simulink model "building_PHPP_v2"  (R2023b)
settings: Solver=ode23s  StartTime=-building.preruntime+8760*3600  StopTime=building.runtime+8760*3600  EnableMultiTasking=on
PreLoadFcn:
  | tic
StartFcn:
  | pre_time = toc
  | assignin('base','pre_time',pre_time)
  | tic
StopFcn:
  | time = toc
  | assignin('base','time',time)
values from neighbouring files (symbols this model uses):
  building = obj    [BUILDING.m]    (also in create_building_automatic.m = building.save(); ini_building_automatic.m = building.add_variant_hvac(building.variant_hvac, hvac); load_building_automatic.m = building.save())
  cp = str2num(value)    [CONSTRUCTION.m]
  p = [timevec_weather weather(:,12)]    [BOUNDARY.m]    (also in WEATHER.m = 0; init_carnotUIBK.m = cell2mat(carnotUIBKpaths(i,2)))
  rho = str2num(value)    [CONSTRUCTION.m]    (also in theta_ground_v1.m = 2000)
undefined symbols (not defined in the file or in its folder): Dreifach, get_building, Qdot_C, Qdot_C_energy, Qdot_H, Qdot_H_energy, Qdot_I_electricity, Qdot_I_electricity_energy, Qdot_I_light, Qdot_I_light_energy, Qdot_I_person, Qdot_I_person_energy, Qdot_S, Qdot_S_energy, Qdot_T_ground, Qdot_T_ground_energy, Qdot_T_neighbour, Qdot_T_neighbour_energy, Qdot_T_opaque, Qdot_T_opaque_energy, Qdot_T_window, Qdot_T_window_energy, Qdot_V_infiltration, Qdot_V_infiltration_energy, Qdot_V_mech, Qdot_V_mech_energy, Qdot_V_window, Qdot_V_window_energy, Tc, Tr, Ts, Wärmeschutzglas, x_CO2, x_H2O, x_VOC
libraries: carnotUIBK x2418, carnot x1
(part 32 of 32)

== system building_PHPP_v2/DATALOGGER/logger_BDB/z4/Subsystem11 ==
  In1 : Inport
  Integrator1 : Integrator
  Ws->kWh : Gain  Gain=1/3600/1000
  Out1 : Outport  VectorParamsAs1DForOutWhenUnconnected=off
  wires:
  Ws->kWh/1 -> Out1/1
  Integrator1/1 -> Ws->kWh/1
  In1/1 -> Integrator1/1

== system building_PHPP_v2/DATALOGGER/logger_BDB/z4/Subsystem12 ==
  In1 : Inport
  Integrator1 : Integrator
  Ws->kWh : Gain  Gain=1/3600/1000
  Out1 : Outport  VectorParamsAs1DForOutWhenUnconnected=off
  wires:
  In1/1 -> Integrator1/1
  Integrator1/1 -> Ws->kWh/1
  Ws->kWh/1 -> Out1/1

== system building_PHPP_v2/DATALOGGER/logger_BDB/z4/Subsystem2 ==
  In1 : Inport
  Integrator1 : Integrator
  Ws->kWh : Gain  Gain=1/3600/1000
  Out1 : Outport  VectorParamsAs1DForOutWhenUnconnected=off
  wires:
  In1/1 -> Integrator1/1
  Integrator1/1 -> Ws->kWh/1
  Ws->kWh/1 -> Out1/1

== system building_PHPP_v2/DATALOGGER/logger_BDB/z4/Subsystem3 ==
  In1 : Inport
  Integrator1 : Integrator
  Ws->kWh : Gain  Gain=1/3600/1000
  Out1 : Outport  VectorParamsAs1DForOutWhenUnconnected=off
  wires:
  Ws->kWh/1 -> Out1/1
  Integrator1/1 -> Ws->kWh/1
  In1/1 -> Integrator1/1

== system building_PHPP_v2/DATALOGGER/logger_BDB/z4/Subsystem4 ==
  In1 : Inport
  Integrator1 : Integrator
  Ws->kWh : Gain  Gain=1/3600/1000
  Out1 : Outport  VectorParamsAs1DForOutWhenUnconnected=off
  wires:
  In1/1 -> Integrator1/1
  Integrator1/1 -> Ws->kWh/1
  Ws->kWh/1 -> Out1/1

== system building_PHPP_v2/DATALOGGER/logger_BDB/z4/Subsystem5 ==
  In1 : Inport
  Integrator1 : Integrator
  Ws->kWh : Gain  Gain=1/3600/1000
  Out1 : Outport  VectorParamsAs1DForOutWhenUnconnected=off
  wires:
  Ws->kWh/1 -> Out1/1
  Integrator1/1 -> Ws->kWh/1
  In1/1 -> Integrator1/1

== system building_PHPP_v2/DATALOGGER/logger_BDB/z4/Subsystem6 ==
  In1 : Inport
  Integrator1 : Integrator
  Ws->kWh : Gain  Gain=1/3600/1000
  Out1 : Outport  VectorParamsAs1DForOutWhenUnconnected=off
  wires:
  In1/1 -> Integrator1/1
  Integrator1/1 -> Ws->kWh/1
  Ws->kWh/1 -> Out1/1

== system building_PHPP_v2/DATALOGGER/logger_BDB/z4/Subsystem7 ==
  In1 : Inport
  Integrator1 : Integrator
  Ws->kWh : Gain  Gain=1/3600/1000
  Out1 : Outport  VectorParamsAs1DForOutWhenUnconnected=off
  wires:
  Ws->kWh/1 -> Out1/1
  Integrator1/1 -> Ws->kWh/1
  In1/1 -> Integrator1/1

== system building_PHPP_v2/DATALOGGER/logger_BDB/z4/Subsystem8 ==
  In1 : Inport
  Integrator1 : Integrator
  Ws->kWh : Gain  Gain=1/3600/1000
  Out1 : Outport  VectorParamsAs1DForOutWhenUnconnected=off
  wires:
  In1/1 -> Integrator1/1
  Integrator1/1 -> Ws->kWh/1
  Ws->kWh/1 -> Out1/1

== system building_PHPP_v2/DATALOGGER/logger_BDB/z4/Subsystem9 ==
  In1 : Inport
  Integrator1 : Integrator
  Ws->kWh : Gain  Gain=1/3600/1000
  Out1 : Outport  VectorParamsAs1DForOutWhenUnconnected=off
  wires:
  Ws->kWh/1 -> Out1/1
  Integrator1/1 -> Ws->kWh/1
  In1/1 -> Integrator1/1

== system building_PHPP_v2/DATALOGGER/logger_BDB/z5/Subsystem ==
  In1 : Inport
  Integrator1 : Integrator
  Ws->kWh : Gain  Gain=1/3600/1000
  Out1 : Outport  VectorParamsAs1DForOutWhenUnconnected=off
  wires:
  Ws->kWh/1 -> Out1/1
  Integrator1/1 -> Ws->kWh/1
  In1/1 -> Integrator1/1

== system building_PHPP_v2/DATALOGGER/logger_BDB/z5/Subsystem1 ==
  In1 : Inport
  Integrator1 : Integrator
  Ws->kWh : Gain  Gain=1/3600/1000
  Out1 : Outport  VectorParamsAs1DForOutWhenUnconnected=off
  wires:
  In1/1 -> Integrator1/1
  Integrator1/1 -> Ws->kWh/1
  Ws->kWh/1 -> Out1/1

== system building_PHPP_v2/DATALOGGER/logger_BDB/z5/Subsystem10 ==
  In1 : Inport
  Integrator1 : Integrator
  Ws->kWh : Gain  Gain=1/3600/1000
  Out1 : Outport  VectorParamsAs1DForOutWhenUnconnected=off
  wires:
  Ws->kWh/1 -> Out1/1
  Integrator1/1 -> Ws->kWh/1
  In1/1 -> Integrator1/1

== system building_PHPP_v2/DATALOGGER/logger_BDB/z5/Subsystem11 ==
  In1 : Inport
  Integrator1 : Integrator
  Ws->kWh : Gain  Gain=1/3600/1000
  Out1 : Outport  VectorParamsAs1DForOutWhenUnconnected=off
  wires:
  In1/1 -> Integrator1/1
  Integrator1/1 -> Ws->kWh/1
  Ws->kWh/1 -> Out1/1

== system building_PHPP_v2/DATALOGGER/logger_BDB/z5/Subsystem12 ==
  In1 : Inport
  Integrator1 : Integrator
  Ws->kWh : Gain  Gain=1/3600/1000
  Out1 : Outport  VectorParamsAs1DForOutWhenUnconnected=off
  wires:
  Ws->kWh/1 -> Out1/1
  Integrator1/1 -> Ws->kWh/1
  In1/1 -> Integrator1/1

== system building_PHPP_v2/DATALOGGER/logger_BDB/z5/Subsystem2 ==
  In1 : Inport
  Integrator1 : Integrator
  Ws->kWh : Gain  Gain=1/3600/1000
  Out1 : Outport  VectorParamsAs1DForOutWhenUnconnected=off
  wires:
  Ws->kWh/1 -> Out1/1
  Integrator1/1 -> Ws->kWh/1
  In1/1 -> Integrator1/1

== system building_PHPP_v2/DATALOGGER/logger_BDB/z5/Subsystem3 ==
  In1 : Inport
  Integrator1 : Integrator
  Ws->kWh : Gain  Gain=1/3600/1000
  Out1 : Outport  VectorParamsAs1DForOutWhenUnconnected=off
  wires:
  In1/1 -> Integrator1/1
  Integrator1/1 -> Ws->kWh/1
  Ws->kWh/1 -> Out1/1

== system building_PHPP_v2/DATALOGGER/logger_BDB/z5/Subsystem4 ==
  In1 : Inport
  Integrator1 : Integrator
  Ws->kWh : Gain  Gain=1/3600/1000
  Out1 : Outport  VectorParamsAs1DForOutWhenUnconnected=off
  wires:
  Ws->kWh/1 -> Out1/1
  Integrator1/1 -> Ws->kWh/1
  In1/1 -> Integrator1/1

== system building_PHPP_v2/DATALOGGER/logger_BDB/z5/Subsystem5 ==
  In1 : Inport
  Integrator1 : Integrator
  Ws->kWh : Gain  Gain=1/3600/1000
  Out1 : Outport  VectorParamsAs1DForOutWhenUnconnected=off
  wires:
  In1/1 -> Integrator1/1
  Integrator1/1 -> Ws->kWh/1
  Ws->kWh/1 -> Out1/1

== system building_PHPP_v2/DATALOGGER/logger_BDB/z5/Subsystem6 ==
  In1 : Inport
  Integrator1 : Integrator
  Ws->kWh : Gain  Gain=1/3600/1000
  Out1 : Outport  VectorParamsAs1DForOutWhenUnconnected=off
  wires:
  Ws->kWh/1 -> Out1/1
  Integrator1/1 -> Ws->kWh/1
  In1/1 -> Integrator1/1

== system building_PHPP_v2/DATALOGGER/logger_BDB/z5/Subsystem7 ==
  In1 : Inport
  Integrator1 : Integrator
  Ws->kWh : Gain  Gain=1/3600/1000
  Out1 : Outport  VectorParamsAs1DForOutWhenUnconnected=off
  wires:
  In1/1 -> Integrator1/1
  Integrator1/1 -> Ws->kWh/1
  Ws->kWh/1 -> Out1/1

== system building_PHPP_v2/DATALOGGER/logger_BDB/z5/Subsystem8 ==
  In1 : Inport
  Integrator1 : Integrator
  Ws->kWh : Gain  Gain=1/3600/1000
  Out1 : Outport  VectorParamsAs1DForOutWhenUnconnected=off
  wires:
  Ws->kWh/1 -> Out1/1
  Integrator1/1 -> Ws->kWh/1
  In1/1 -> Integrator1/1

== system building_PHPP_v2/DATALOGGER/logger_BDB/z5/Subsystem9 ==
  In1 : Inport
  Integrator1 : Integrator
  Ws->kWh : Gain  Gain=1/3600/1000
  Out1 : Outport  VectorParamsAs1DForOutWhenUnconnected=off
  wires:
  In1/1 -> Integrator1/1
  Integrator1/1 -> Ws->kWh/1
  Ws->kWh/1 -> Out1/1

== system building_PHPP_v2/DATALOGGER/logger_BDB/z6/Subsystem ==
  In1 : Inport
  Integrator1 : Integrator
  Ws->kWh : Gain  Gain=1/3600/1000
  Out1 : Outport  VectorParamsAs1DForOutWhenUnconnected=off
  wires:
  In1/1 -> Integrator1/1
  Integrator1/1 -> Ws->kWh/1
  Ws->kWh/1 -> Out1/1

== system building_PHPP_v2/DATALOGGER/logger_BDB/z6/Subsystem1 ==
  In1 : Inport
  Integrator1 : Integrator
  Ws->kWh : Gain  Gain=1/3600/1000
  Out1 : Outport  VectorParamsAs1DForOutWhenUnconnected=off
  wires:
  Ws->kWh/1 -> Out1/1
  Integrator1/1 -> Ws->kWh/1
  In1/1 -> Integrator1/1

== system building_PHPP_v2/DATALOGGER/logger_BDB/z6/Subsystem10 ==
  In1 : Inport
  Integrator1 : Integrator
  Ws->kWh : Gain  Gain=1/3600/1000
  Out1 : Outport  VectorParamsAs1DForOutWhenUnconnected=off
  wires:
  In1/1 -> Integrator1/1
  Integrator1/1 -> Ws->kWh/1
  Ws->kWh/1 -> Out1/1

== system building_PHPP_v2/DATALOGGER/logger_BDB/z6/Subsystem11 ==
  In1 : Inport
  Integrator1 : Integrator
  Ws->kWh : Gain  Gain=1/3600/1000
  Out1 : Outport  VectorParamsAs1DForOutWhenUnconnected=off
  wires:
  Ws->kWh/1 -> Out1/1
  Integrator1/1 -> Ws->kWh/1
  In1/1 -> Integrator1/1

== system building_PHPP_v2/DATALOGGER/logger_BDB/z6/Subsystem12 ==
  In1 : Inport
  Integrator1 : Integrator
  Ws->kWh : Gain  Gain=1/3600/1000
  Out1 : Outport  VectorParamsAs1DForOutWhenUnconnected=off
  wires:
  In1/1 -> Integrator1/1
  Integrator1/1 -> Ws->kWh/1
  Ws->kWh/1 -> Out1/1

== system building_PHPP_v2/DATALOGGER/logger_BDB/z6/Subsystem2 ==
  In1 : Inport
  Integrator1 : Integrator
  Ws->kWh : Gain  Gain=1/3600/1000
  Out1 : Outport  VectorParamsAs1DForOutWhenUnconnected=off
  wires:
  In1/1 -> Integrator1/1
  Integrator1/1 -> Ws->kWh/1
  Ws->kWh/1 -> Out1/1

== system building_PHPP_v2/DATALOGGER/logger_BDB/z6/Subsystem3 ==
  In1 : Inport
  Integrator1 : Integrator
  Ws->kWh : Gain  Gain=1/3600/1000
  Out1 : Outport  VectorParamsAs1DForOutWhenUnconnected=off
  wires:
  Ws->kWh/1 -> Out1/1
  Integrator1/1 -> Ws->kWh/1
  In1/1 -> Integrator1/1

== system building_PHPP_v2/DATALOGGER/logger_BDB/z6/Subsystem4 ==
  In1 : Inport
  Integrator1 : Integrator
  Ws->kWh : Gain  Gain=1/3600/1000
  Out1 : Outport  VectorParamsAs1DForOutWhenUnconnected=off
  wires:
  In1/1 -> Integrator1/1
  Integrator1/1 -> Ws->kWh/1
  Ws->kWh/1 -> Out1/1

== system building_PHPP_v2/DATALOGGER/logger_BDB/z6/Subsystem5 ==
  In1 : Inport
  Integrator1 : Integrator
  Ws->kWh : Gain  Gain=1/3600/1000
  Out1 : Outport  VectorParamsAs1DForOutWhenUnconnected=off
  wires:
  Ws->kWh/1 -> Out1/1
  Integrator1/1 -> Ws->kWh/1
  In1/1 -> Integrator1/1

== system building_PHPP_v2/DATALOGGER/logger_BDB/z6/Subsystem6 ==
  In1 : Inport
  Integrator1 : Integrator
  Ws->kWh : Gain  Gain=1/3600/1000
  Out1 : Outport  VectorParamsAs1DForOutWhenUnconnected=off
  wires:
  In1/1 -> Integrator1/1
  Integrator1/1 -> Ws->kWh/1
  Ws->kWh/1 -> Out1/1

== system building_PHPP_v2/DATALOGGER/logger_BDB/z6/Subsystem7 ==
  In1 : Inport
  Integrator1 : Integrator
  Ws->kWh : Gain  Gain=1/3600/1000
  Out1 : Outport  VectorParamsAs1DForOutWhenUnconnected=off
  wires:
  Ws->kWh/1 -> Out1/1
  Integrator1/1 -> Ws->kWh/1
  In1/1 -> Integrator1/1

== system building_PHPP_v2/DATALOGGER/logger_BDB/z6/Subsystem8 ==
  In1 : Inport
  Integrator1 : Integrator
  Ws->kWh : Gain  Gain=1/3600/1000
  Out1 : Outport  VectorParamsAs1DForOutWhenUnconnected=off
  wires:
  In1/1 -> Integrator1/1
  Integrator1/1 -> Ws->kWh/1
  Ws->kWh/1 -> Out1/1

== system building_PHPP_v2/DATALOGGER/logger_BDB/z6/Subsystem9 ==
  In1 : Inport
  Integrator1 : Integrator
  Ws->kWh : Gain  Gain=1/3600/1000
  Out1 : Outport  VectorParamsAs1DForOutWhenUnconnected=off
  wires:
  Ws->kWh/1 -> Out1/1
  Integrator1/1 -> Ws->kWh/1
  In1/1 -> Integrator1/1

== system building_PHPP_v2/DATALOGGER/logger_BDB/z7/Subsystem ==
  In1 : Inport
  Integrator1 : Integrator
  Ws->kWh : Gain  Gain=1/3600/1000
  Out1 : Outport  VectorParamsAs1DForOutWhenUnconnected=off
  wires:
  Ws->kWh/1 -> Out1/1
  Integrator1/1 -> Ws->kWh/1
  In1/1 -> Integrator1/1

== system building_PHPP_v2/DATALOGGER/logger_BDB/z7/Subsystem1 ==
  In1 : Inport
  Integrator1 : Integrator
  Ws->kWh : Gain  Gain=1/3600/1000
  Out1 : Outport  VectorParamsAs1DForOutWhenUnconnected=off
  wires:
  In1/1 -> Integrator1/1
  Integrator1/1 -> Ws->kWh/1
  Ws->kWh/1 -> Out1/1

== system building_PHPP_v2/DATALOGGER/logger_BDB/z7/Subsystem10 ==
  In1 : Inport
  Integrator1 : Integrator
  Ws->kWh : Gain  Gain=1/3600/1000
  Out1 : Outport  VectorParamsAs1DForOutWhenUnconnected=off
  wires:
  Ws->kWh/1 -> Out1/1
  Integrator1/1 -> Ws->kWh/1
  In1/1 -> Integrator1/1

== system building_PHPP_v2/DATALOGGER/logger_BDB/z7/Subsystem11 ==
  In1 : Inport
  Integrator1 : Integrator
  Ws->kWh : Gain  Gain=1/3600/1000
  Out1 : Outport  VectorParamsAs1DForOutWhenUnconnected=off
  wires:
  In1/1 -> Integrator1/1
  Integrator1/1 -> Ws->kWh/1
  Ws->kWh/1 -> Out1/1

== system building_PHPP_v2/DATALOGGER/logger_BDB/z7/Subsystem12 ==
  In1 : Inport
  Integrator1 : Integrator
  Ws->kWh : Gain  Gain=1/3600/1000
  Out1 : Outport  VectorParamsAs1DForOutWhenUnconnected=off
  wires:
  Ws->kWh/1 -> Out1/1
  Integrator1/1 -> Ws->kWh/1
  In1/1 -> Integrator1/1

== system building_PHPP_v2/DATALOGGER/logger_BDB/z7/Subsystem2 ==
  In1 : Inport
  Integrator1 : Integrator
  Ws->kWh : Gain  Gain=1/3600/1000
  Out1 : Outport  VectorParamsAs1DForOutWhenUnconnected=off
  wires:
  Ws->kWh/1 -> Out1/1
  Integrator1/1 -> Ws->kWh/1
  In1/1 -> Integrator1/1

== system building_PHPP_v2/DATALOGGER/logger_BDB/z7/Subsystem3 ==
  In1 : Inport
  Integrator1 : Integrator
  Ws->kWh : Gain  Gain=1/3600/1000
  Out1 : Outport  VectorParamsAs1DForOutWhenUnconnected=off
  wires:
  In1/1 -> Integrator1/1
  Integrator1/1 -> Ws->kWh/1
  Ws->kWh/1 -> Out1/1

== system building_PHPP_v2/DATALOGGER/logger_BDB/z7/Subsystem4 ==
  In1 : Inport
  Integrator1 : Integrator
  Ws->kWh : Gain  Gain=1/3600/1000
  Out1 : Outport  VectorParamsAs1DForOutWhenUnconnected=off
  wires:
  Ws->kWh/1 -> Out1/1
  Integrator1/1 -> Ws->kWh/1
  In1/1 -> Integrator1/1

== system building_PHPP_v2/DATALOGGER/logger_BDB/z7/Subsystem5 ==
  In1 : Inport
  Integrator1 : Integrator
  Ws->kWh : Gain  Gain=1/3600/1000
  Out1 : Outport  VectorParamsAs1DForOutWhenUnconnected=off
  wires:
  In1/1 -> Integrator1/1
  Integrator1/1 -> Ws->kWh/1
  Ws->kWh/1 -> Out1/1

== system building_PHPP_v2/DATALOGGER/logger_BDB/z7/Subsystem6 ==
  In1 : Inport
  Integrator1 : Integrator
  Ws->kWh : Gain  Gain=1/3600/1000
  Out1 : Outport  VectorParamsAs1DForOutWhenUnconnected=off
  wires:
  Ws->kWh/1 -> Out1/1
  Integrator1/1 -> Ws->kWh/1
  In1/1 -> Integrator1/1

== system building_PHPP_v2/DATALOGGER/logger_BDB/z7/Subsystem7 ==
  In1 : Inport
  Integrator1 : Integrator
  Ws->kWh : Gain  Gain=1/3600/1000
  Out1 : Outport  VectorParamsAs1DForOutWhenUnconnected=off
  wires:
  In1/1 -> Integrator1/1
  Integrator1/1 -> Ws->kWh/1
  Ws->kWh/1 -> Out1/1

== system building_PHPP_v2/DATALOGGER/logger_BDB/z7/Subsystem8 ==
  In1 : Inport
  Integrator1 : Integrator
  Ws->kWh : Gain  Gain=1/3600/1000
  Out1 : Outport  VectorParamsAs1DForOutWhenUnconnected=off
  wires:
  Ws->kWh/1 -> Out1/1
  Integrator1/1 -> Ws->kWh/1
  In1/1 -> Integrator1/1

== system building_PHPP_v2/DATALOGGER/logger_BDB/z7/Subsystem9 ==
  In1 : Inport
  Integrator1 : Integrator
  Ws->kWh : Gain  Gain=1/3600/1000
  Out1 : Outport  VectorParamsAs1DForOutWhenUnconnected=off
  wires:
  In1/1 -> Integrator1/1
  Integrator1/1 -> Ws->kWh/1
  Ws->kWh/1 -> Out1/1

== system building_PHPP_v2/DATALOGGER/logger_BDB/z8/Subsystem ==
  In1 : Inport
  Integrator1 : Integrator
  Ws->kWh : Gain  Gain=1/3600/1000
  Out1 : Outport  VectorParamsAs1DForOutWhenUnconnected=off
  wires:
  In1/1 -> Integrator1/1
  Integrator1/1 -> Ws->kWh/1
  Ws->kWh/1 -> Out1/1

== system building_PHPP_v2/DATALOGGER/logger_BDB/z8/Subsystem1 ==
  In1 : Inport
  Integrator1 : Integrator
  Ws->kWh : Gain  Gain=1/3600/1000
  Out1 : Outport  VectorParamsAs1DForOutWhenUnconnected=off
  wires:
  Ws->kWh/1 -> Out1/1
  Integrator1/1 -> Ws->kWh/1
  In1/1 -> Integrator1/1

== system building_PHPP_v2/DATALOGGER/logger_BDB/z8/Subsystem10 ==
  In1 : Inport
  Integrator1 : Integrator
  Ws->kWh : Gain  Gain=1/3600/1000
  Out1 : Outport  VectorParamsAs1DForOutWhenUnconnected=off
  wires:
  In1/1 -> Integrator1/1
  Integrator1/1 -> Ws->kWh/1
  Ws->kWh/1 -> Out1/1

== system building_PHPP_v2/DATALOGGER/logger_BDB/z8/Subsystem11 ==
  In1 : Inport
  Integrator1 : Integrator
  Ws->kWh : Gain  Gain=1/3600/1000
  Out1 : Outport  VectorParamsAs1DForOutWhenUnconnected=off
  wires:
  Ws->kWh/1 -> Out1/1
  Integrator1/1 -> Ws->kWh/1
  In1/1 -> Integrator1/1

== system building_PHPP_v2/DATALOGGER/logger_BDB/z8/Subsystem12 ==
  In1 : Inport
  Integrator1 : Integrator
  Ws->kWh : Gain  Gain=1/3600/1000
  Out1 : Outport  VectorParamsAs1DForOutWhenUnconnected=off
  wires:
  In1/1 -> Integrator1/1
  Integrator1/1 -> Ws->kWh/1
  Ws->kWh/1 -> Out1/1

== system building_PHPP_v2/DATALOGGER/logger_BDB/z8/Subsystem2 ==
  In1 : Inport
  Integrator1 : Integrator
  Ws->kWh : Gain  Gain=1/3600/1000
  Out1 : Outport  VectorParamsAs1DForOutWhenUnconnected=off
  wires:
  In1/1 -> Integrator1/1
  Integrator1/1 -> Ws->kWh/1
  Ws->kWh/1 -> Out1/1

== system building_PHPP_v2/DATALOGGER/logger_BDB/z8/Subsystem3 ==
  In1 : Inport
  Integrator1 : Integrator
  Ws->kWh : Gain  Gain=1/3600/1000
  Out1 : Outport  VectorParamsAs1DForOutWhenUnconnected=off
  wires:
  Ws->kWh/1 -> Out1/1
  Integrator1/1 -> Ws->kWh/1
  In1/1 -> Integrator1/1

== system building_PHPP_v2/DATALOGGER/logger_BDB/z8/Subsystem4 ==
  In1 : Inport
  Integrator1 : Integrator
  Ws->kWh : Gain  Gain=1/3600/1000
  Out1 : Outport  VectorParamsAs1DForOutWhenUnconnected=off
  wires:
  In1/1 -> Integrator1/1
  Integrator1/1 -> Ws->kWh/1
  Ws->kWh/1 -> Out1/1

== system building_PHPP_v2/DATALOGGER/logger_BDB/z8/Subsystem5 ==
  In1 : Inport
  Integrator1 : Integrator
  Ws->kWh : Gain  Gain=1/3600/1000
  Out1 : Outport  VectorParamsAs1DForOutWhenUnconnected=off
  wires:
  Ws->kWh/1 -> Out1/1
  Integrator1/1 -> Ws->kWh/1
  In1/1 -> Integrator1/1

== system building_PHPP_v2/DATALOGGER/logger_BDB/z8/Subsystem6 ==
  In1 : Inport
  Integrator1 : Integrator
  Ws->kWh : Gain  Gain=1/3600/1000
  Out1 : Outport  VectorParamsAs1DForOutWhenUnconnected=off
  wires:
  In1/1 -> Integrator1/1
  Integrator1/1 -> Ws->kWh/1
  Ws->kWh/1 -> Out1/1

== system building_PHPP_v2/DATALOGGER/logger_BDB/z8/Subsystem7 ==
  In1 : Inport
  Integrator1 : Integrator
  Ws->kWh : Gain  Gain=1/3600/1000
  Out1 : Outport  VectorParamsAs1DForOutWhenUnconnected=off
  wires:
  Ws->kWh/1 -> Out1/1
  Integrator1/1 -> Ws->kWh/1
  In1/1 -> Integrator1/1

== system building_PHPP_v2/DATALOGGER/logger_BDB/z8/Subsystem8 ==
  In1 : Inport
  Integrator1 : Integrator
  Ws->kWh : Gain  Gain=1/3600/1000
  Out1 : Outport  VectorParamsAs1DForOutWhenUnconnected=off
  wires:
  In1/1 -> Integrator1/1
  Integrator1/1 -> Ws->kWh/1
  Ws->kWh/1 -> Out1/1

== system building_PHPP_v2/DATALOGGER/logger_BDB/z8/Subsystem9 ==
  In1 : Inport
  Integrator1 : Integrator
  Ws->kWh : Gain  Gain=1/3600/1000
  Out1 : Outport  VectorParamsAs1DForOutWhenUnconnected=off
  wires:
  Ws->kWh/1 -> Out1/1
  Integrator1/1 -> Ws->kWh/1
  In1/1 -> Integrator1/1

== system building_PHPP_v2/DATALOGGER/logger_BDB/z9/Subsystem ==
  In1 : Inport
  Integrator1 : Integrator
  Ws->kWh : Gain  Gain=1/3600/1000
  Out1 : Outport  VectorParamsAs1DForOutWhenUnconnected=off
  wires:
  Ws->kWh/1 -> Out1/1
  Integrator1/1 -> Ws->kWh/1
  In1/1 -> Integrator1/1

== system building_PHPP_v2/DATALOGGER/logger_BDB/z9/Subsystem1 ==
  In1 : Inport
  Integrator1 : Integrator
  Ws->kWh : Gain  Gain=1/3600/1000
  Out1 : Outport  VectorParamsAs1DForOutWhenUnconnected=off
  wires:
  In1/1 -> Integrator1/1
  Integrator1/1 -> Ws->kWh/1
  Ws->kWh/1 -> Out1/1

== system building_PHPP_v2/DATALOGGER/logger_BDB/z9/Subsystem10 ==
  In1 : Inport
  Integrator1 : Integrator
  Ws->kWh : Gain  Gain=1/3600/1000
  Out1 : Outport  VectorParamsAs1DForOutWhenUnconnected=off
  wires:
  Ws->kWh/1 -> Out1/1
  Integrator1/1 -> Ws->kWh/1
  In1/1 -> Integrator1/1

== system building_PHPP_v2/DATALOGGER/logger_BDB/z9/Subsystem11 ==
  In1 : Inport
  Integrator1 : Integrator
  Ws->kWh : Gain  Gain=1/3600/1000
  Out1 : Outport  VectorParamsAs1DForOutWhenUnconnected=off
  wires:
  In1/1 -> Integrator1/1
  Integrator1/1 -> Ws->kWh/1
  Ws->kWh/1 -> Out1/1

== system building_PHPP_v2/DATALOGGER/logger_BDB/z9/Subsystem12 ==
  In1 : Inport
  Integrator1 : Integrator
  Ws->kWh : Gain  Gain=1/3600/1000
  Out1 : Outport  VectorParamsAs1DForOutWhenUnconnected=off
  wires:
  Ws->kWh/1 -> Out1/1
  Integrator1/1 -> Ws->kWh/1
  In1/1 -> Integrator1/1

== system building_PHPP_v2/DATALOGGER/logger_BDB/z9/Subsystem2 ==
  In1 : Inport
  Integrator1 : Integrator
  Ws->kWh : Gain  Gain=1/3600/1000
  Out1 : Outport  VectorParamsAs1DForOutWhenUnconnected=off
  wires:
  Ws->kWh/1 -> Out1/1
  Integrator1/1 -> Ws->kWh/1
  In1/1 -> Integrator1/1

== system building_PHPP_v2/DATALOGGER/logger_BDB/z9/Subsystem3 ==
  In1 : Inport
  Integrator1 : Integrator
  Ws->kWh : Gain  Gain=1/3600/1000
  Out1 : Outport  VectorParamsAs1DForOutWhenUnconnected=off
  wires:
  In1/1 -> Integrator1/1
  Integrator1/1 -> Ws->kWh/1
  Ws->kWh/1 -> Out1/1

== system building_PHPP_v2/DATALOGGER/logger_BDB/z9/Subsystem4 ==
  In1 : Inport
  Integrator1 : Integrator
  Ws->kWh : Gain  Gain=1/3600/1000
  Out1 : Outport  VectorParamsAs1DForOutWhenUnconnected=off
  wires:
  Ws->kWh/1 -> Out1/1
  Integrator1/1 -> Ws->kWh/1
  In1/1 -> Integrator1/1

== system building_PHPP_v2/DATALOGGER/logger_BDB/z9/Subsystem5 ==
  In1 : Inport
  Integrator1 : Integrator
  Ws->kWh : Gain  Gain=1/3600/1000
  Out1 : Outport  VectorParamsAs1DForOutWhenUnconnected=off
  wires:
  In1/1 -> Integrator1/1
  Integrator1/1 -> Ws->kWh/1
  Ws->kWh/1 -> Out1/1

== system building_PHPP_v2/DATALOGGER/logger_BDB/z9/Subsystem6 ==
  In1 : Inport
  Integrator1 : Integrator
  Ws->kWh : Gain  Gain=1/3600/1000
  Out1 : Outport  VectorParamsAs1DForOutWhenUnconnected=off
  wires:
  Ws->kWh/1 -> Out1/1
  Integrator1/1 -> Ws->kWh/1
  In1/1 -> Integrator1/1

== system building_PHPP_v2/DATALOGGER/logger_BDB/z9/Subsystem7 ==
  In1 : Inport
  Integrator1 : Integrator
  Ws->kWh : Gain  Gain=1/3600/1000
  Out1 : Outport  VectorParamsAs1DForOutWhenUnconnected=off
  wires:
  In1/1 -> Integrator1/1
  Integrator1/1 -> Ws->kWh/1
  Ws->kWh/1 -> Out1/1

== system building_PHPP_v2/DATALOGGER/logger_BDB/z9/Subsystem8 ==
  In1 : Inport
  Integrator1 : Integrator
  Ws->kWh : Gain  Gain=1/3600/1000
  Out1 : Outport  VectorParamsAs1DForOutWhenUnconnected=off
  wires:
  Ws->kWh/1 -> Out1/1
  Integrator1/1 -> Ws->kWh/1
  In1/1 -> Integrator1/1

== system building_PHPP_v2/DATALOGGER/logger_BDB/z9/Subsystem9 ==
  In1 : Inport
  Integrator1 : Integrator
  Ws->kWh : Gain  Gain=1/3600/1000
  Out1 : Outport  VectorParamsAs1DForOutWhenUnconnected=off
  wires:
  In1/1 -> Integrator1/1
  Integrator1/1 -> Ws->kWh/1
  Ws->kWh/1 -> Out1/1
